simulink model "Adaptive_cruise_control_01"  (R2020a)
settings: Solver=VariableStepAuto  StartTime=0.0  StopTime=100  RelTol=1e-3
libraries: simulink x4, vrlib x2, mpcadaslib x1, robotmobilelib x1, autolibshared x1
settings Model: Creator=NIKHIL  LastModifiedBy=NIKHIL

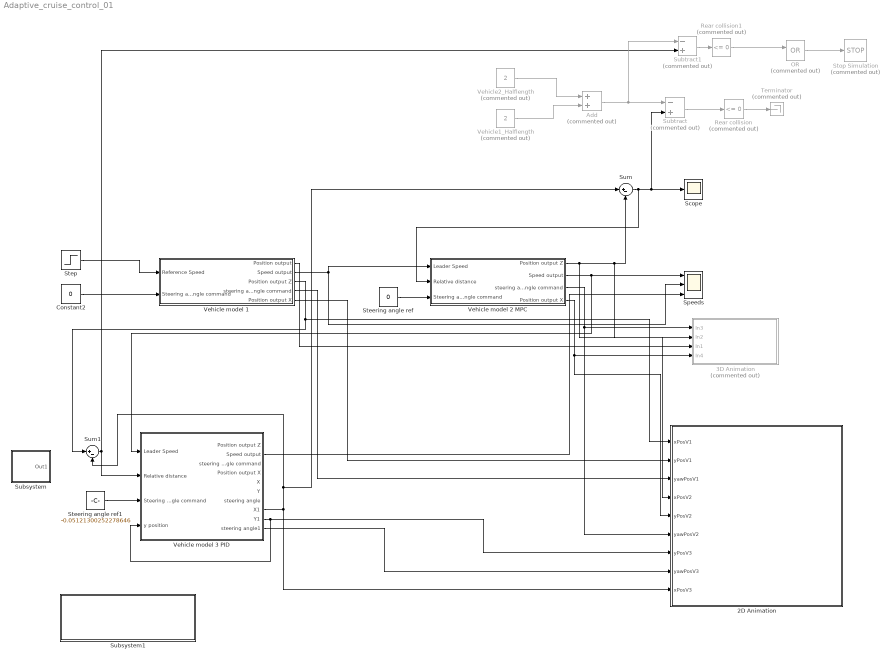
== system Adaptive_cruise_control_01 ==
  2D Animation : Subsystem  TreatAsAtomicUnit=on  SystemSampleTime=0.02
  3D Animation : Subsystem  Commented=on
  Add : Sum  Commented=on
  Constant2 : Constant  Value=0
  OR : Logic  Commented=on  Operator=OR  IconShape=distinctive  AllPortsSameDT=off  OutDataTypeStr=boolean
  Rear collision : simulink/Logic and Bit Operations/Compare To Constant  Commented=on  relop=<=  const=0  OutDataTypeStr=boolean
  Rear collision1 : simulink/Logic and Bit Operations/Compare To Constant  Commented=on  relop=<=  const=0  OutDataTypeStr=boolean
  Scope : Scope
  "Speeds " : Scope  NumInputPorts=3
  Steering angle ref : Constant  Value=0
  Steering angle ref1 : Constant  Value=-0.05121300252278646
  Step : Step  Time=10.5  Before=8  After=8  SampleTime=0
  Stop Simulation : Stop  Commented=on
  Subsystem : Subsystem
  Subsystem1 : Subsystem
  Subtract : Sum  Commented=on  Inputs=-+
  Subtract1 : Sum  Commented=on  Inputs=-+
  Sum : Sum  Inputs=|+-
  Sum1 : Sum  Inputs=|+-
  Terminator : Terminator  Commented=on
  Vehicle model 1 : Subsystem  mask{Pos=10, Speed=25}
      mask prompts: Pos "Initial position"; Speed "Initial speed"
      mask TypeOptions Pos: Initial position Z/Value
      mask TypeOptions Speed: Initial speed/Value
  Vehicle model 2 MPC : Subsystem  mask{Pos=50, Speed=25}
      mask prompts: Pos "Initial position"; Speed "Initial speed"
      mask TypeOptions Pos: Initial position Z/Value
      mask TypeOptions Speed: Initial speed/Value
  Vehicle model 3 PID : Subsystem  mask{Pos=0, Speed=45}
      mask prompts: Pos "Initial position"; Speed "Initial speed"
      mask TypeOptions Pos: Initial position Z/Value
      mask TypeOptions Speed: Initial speed/Value
  Vehicle1_Halflength : Constant  Commented=on  Value=2
  Vehicle2_Halflength : Constant  Commented=on  Value=2
  wires:
  Vehicle model 2 MPC/3(steering angle command) -> 2D Animation/6(yawPosV2), 3D Animation/1(In3)
  Sum1/1 -> Vehicle model 3 PID/2(Relative distance), Subtract1/2
  Subtract1/1 -> Rear collision1/1
  Vehicle model 3 PID/9(Y1) -> Vehicle model 3 PID/4(y position), 2D Animation/7(yPosV3)
  Subtract/1 -> Rear collision/1
  Vehicle model 3 PID/2(Speed output) -> "Speeds "/3
  Vehicle model 3 PID/8(X1) -> Sum/1, Sum1/2, 2D Animation/9(xPosV3)
  Vehicle model 3 PID/10(steering angle1) -> 2D Animation/8(yawPosV3)
  Sum/1 -> Vehicle model 2 MPC/2(Relative distance), Subtract/2, Scope/1
  Steering angle ref/1 -> Vehicle model 2 MPC/3(Steering angle command)
  Vehicle model 2 MPC/2(Speed output) -> Vehicle model 3 PID/1(Leader Speed), "Speeds "/1
  OR/1 -> Stop Simulation/1
  Vehicle model 2 MPC/1(Position output Z) -> 2D Animation/4(xPosV2), Sum/2, 3D Animation/2(In2)
  Add/1 -> Subtract1/1, Subtract/1
  Vehicle2_Halflength/1 -> Add/1
  Vehicle model 1/1(Position output) -> 3D Animation/3(In1)
  Vehicle1_Halflength/1 -> Add/2
  Vehicle model 1/2(Speed output) -> "Speeds "/2, Vehicle model 2 MPC/1(Leader Speed)
  Vehicle model 2 MPC/4(Position output X) -> 2D Animation/5(yPosV2), 3D Animation/4(In4)
  Constant2/1 -> Vehicle model 1/2(Steering angle command)
  Vehicle model 1/3(Position output Z) -> 2D Animation/1(xPosV1), Sum1/1
  Steering angle ref1/1 -> Vehicle model 3 PID/3(Steering angle command)
  Rear collision1/1 -> OR/1
  Rear collision/1 -> Terminator/1
  Vehicle model 1/5(Position output X) -> 2D Animation/2(yPosV1)
  Vehicle model 1/4(steering angle command) -> 2D Animation/3(yawPosV1)
  Step/1 -> Vehicle model 1/1(Reference Speed)

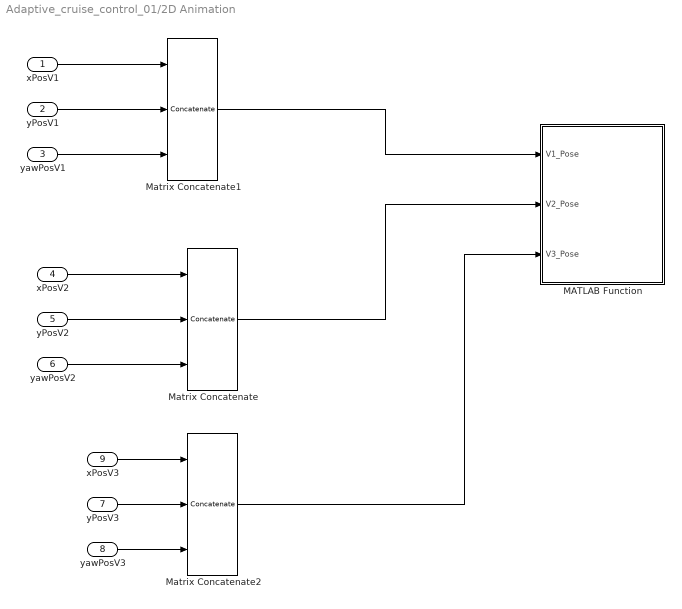
== system Adaptive_cruise_control_01/2D Animation ==
  xPosV1 : Inport
  yPosV1 : Inport  Port=2
  yawPosV1 : Inport  Port=3
  xPosV2 : Inport  Port=4
  yPosV2 : Inport  Port=5
  yawPosV2 : Inport  Port=6
  yPosV3 : Inport  Port=7
  yawPosV3 : Inport  Port=8
  xPosV3 : Inport  Port=9
  MATLAB Function : MATLAB Function  TreatAsAtomicUnit=on
      mask init:
      | close all;
      | figure('units','normalized','outerposition',[0 0 1 1]);
      | grid on
      | axis equal
      | hold on
  Matrix Concatenate : Concatenate  NumInputs=3  ConcatenateDimension=2
  Matrix Concatenate1 : Concatenate  NumInputs=3  ConcatenateDimension=2
  Matrix Concatenate2 : Concatenate  NumInputs=3  ConcatenateDimension=2
  wires:
  xPosV2/1 -> Matrix Concatenate/1
  yPosV2/1 -> Matrix Concatenate/2
  yawPosV2/1 -> Matrix Concatenate/3
  Matrix Concatenate/1 -> MATLAB Function/2(V2_Pose)
  xPosV1/1 -> Matrix Concatenate1/1
  yPosV1/1 -> Matrix Concatenate1/2
  yawPosV1/1 -> Matrix Concatenate1/3
  Matrix Concatenate1/1 -> MATLAB Function/1(V1_Pose)
  xPosV3/1 -> Matrix Concatenate2/1
  yPosV3/1 -> Matrix Concatenate2/2
  yawPosV3/1 -> Matrix Concatenate2/3
  Matrix Concatenate2/1 -> MATLAB Function/3(V3_Pose)

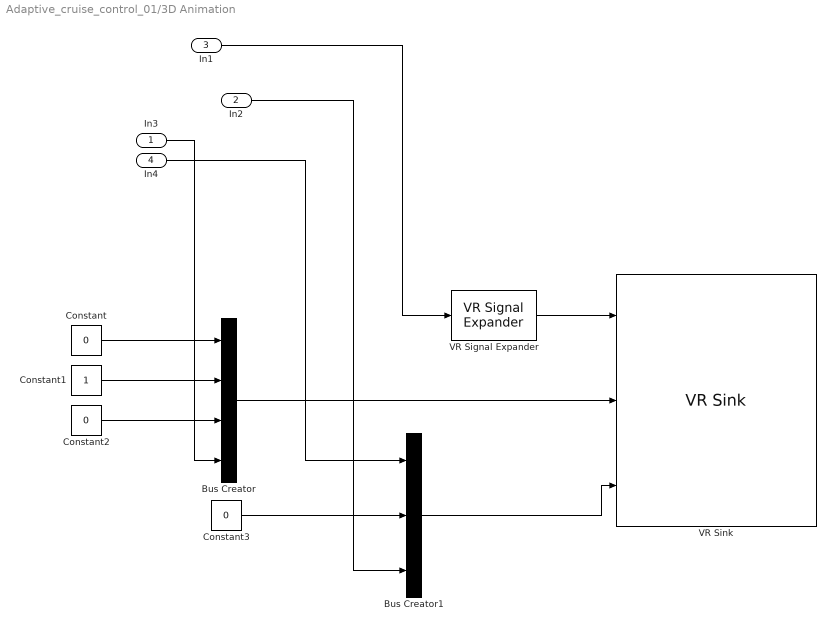
== system Adaptive_cruise_control_01/3D Animation ==
  In3 : Inport
  In2 : Inport  Port=2
  In1 : Inport  Port=3
  In4 : Inport  Port=4
  Bus Creator : BusCreator  Inputs=4
  Bus Creator1 : BusCreator  Inputs=3
  Constant : Constant  Value=0
  Constant1 : Constant
  Constant2 : Constant  Value=0
  Constant3 : Constant  Value=0
  VR Signal Expander : vrlib/VR Signal Expander  outwidth=3  outidx=[3]
  VR Sink : vrlib/VR Sink  InstantiateOnLoad=on  SampleTime=0.02  ViewEnable=on  RemoteChange=off  RemoteView=off  FieldsWritten=Car_Red.translation.3.1.1.double#Car_Blue.rotation.4.1.1.double#Car_Blue.translation.3.1.1.double  WorldFileName=PlatoonWorld.WRL  AutoView=off  VideoDimensions=[]  AllowVariableSize=off
  wires:
  In2/1 -> Bus Creator1/3
  Constant2/1 -> Bus Creator/3
  VR Signal Expander/1 -> VR Sink/1
  Bus Creator/1 -> VR Sink/2
  Constant1/1 -> Bus Creator/2
  Constant/1 -> Bus Creator/1
  Bus Creator1/1 -> VR Sink/3
  In4/1 -> Bus Creator1/1
  Constant3/1 -> Bus Creator1/2
  In1/1 -> VR Signal Expander/1
  In3/1 -> Bus Creator/4

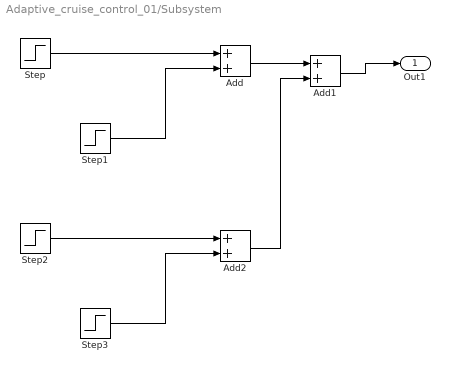
== system Adaptive_cruise_control_01/Subsystem ==
  Add : Sum
  Add1 : Sum
  Add2 : Sum
  Step : Step  Time=0  After=0.2  SampleTime=0
  Step1 : Step  After=-0.2  SampleTime=0
  Step2 : Step  Time=5  After=-0.12  SampleTime=0
  Step3 : Step  Time=6  After=0.12  SampleTime=0
  Out1 : Outport
  wires:
  Add/1 -> Add1/1
  Step/1 -> Add/1
  Step1/1 -> Add/2
  Step3/1 -> Add2/2
  Step2/1 -> Add2/1
  Add2/1 -> Add1/2
  Add1/1 -> Out1/1

== system Adaptive_cruise_control_01/Subsystem1 ==
  Dashboard Scope : DashboardScope
  Gauge : CircularGaugeBlock
  Knob : KnobBlock  ScaleMin=-0.2  ScaleMax=0.2

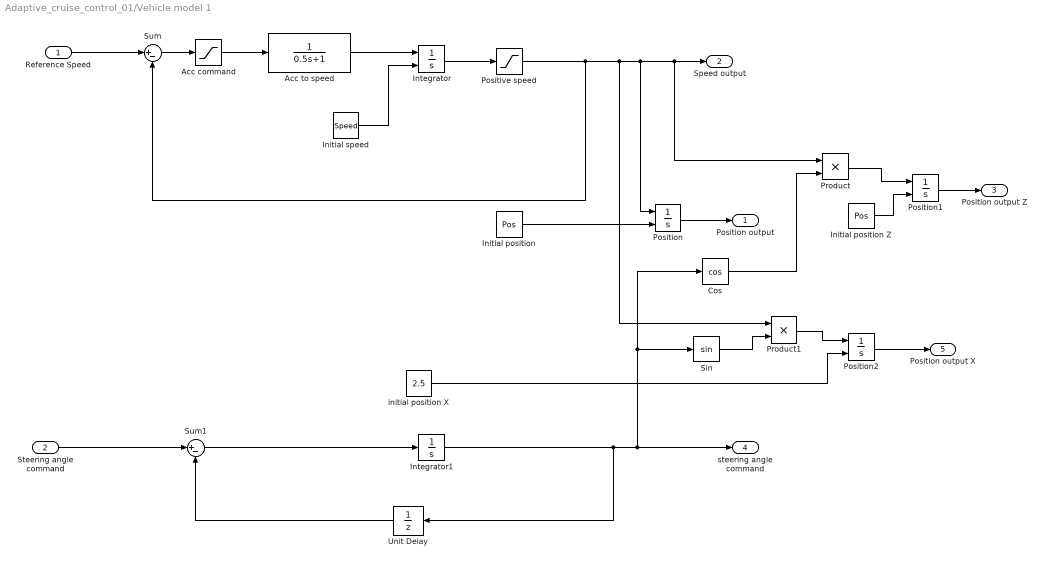
== system Adaptive_cruise_control_01/Vehicle model 1 ==
  Reference Speed : Inport
  Steering angle command : Inport  Port=2
  Acc command : Saturate  UpperLimit=2  LowerLimit=-3
  Acc to speed : TransferFcn  Denominator=[0.5 1]
  Cos : Trigonometry  Operator=cos
  Initial position : Constant  Value=Pos
  Initial position Z : Constant  Value=Pos
  Initial speed : Constant  Value=Speed
  Integrator : Integrator  InitialConditionSource=external
  Integrator1 : Integrator
  Position : Integrator  InitialConditionSource=external
  Position1 : Integrator  InitialConditionSource=external
  Position2 : Integrator  InitialConditionSource=external
  Positive speed : Saturate  UpperLimit=inf
  Product : Product
  Product1 : Product
  Sin : Trigonometry
  Sum : Sum  Inputs=|+-
  Sum1 : Sum  Inputs=|+-
  Unit Delay : UnitDelay  SampleTime=-1  HasFrameUpgradeWarning=on
  initial position X : Constant  Value=2.5
  Position output : Outport
  Speed output : Outport  Port=2
  Position output Z : Outport  Port=3
  steering angle command : Outport  Port=4
  Position output X : Outport  Port=5
  wires:
  Initial speed/1 -> Integrator/2
  Initial position/1 -> Position/2
  Sum/1 -> Acc command/1
  Integrator/1 -> Positive speed/1
  Acc to speed/1 -> Integrator/1
  Acc command/1 -> Acc to speed/1
  Position/1 -> Position output/1
  Reference Speed/1 -> Sum/1
  Cos/1 -> Product/2
  Initial position Z/1 -> Position1/2
  Product/1 -> Position1/1
  Position1/1 -> Position output Z/1
  Unit Delay/1 -> Sum1/2
  Position2/1 -> Position output X/1
  initial position X/1 -> Position2/2
  Sin/1 -> Product1/2
  Product1/1 -> Position2/1
  Integrator1/1 -> steering angle command/1, Sin/1, Cos/1, Unit Delay/1
  Steering angle command/1 -> Sum1/1
  Positive speed/1 -> Product1/1, Product/1, Speed output/1, Position/1, Sum/2
  Sum1/1 -> Integrator1/1

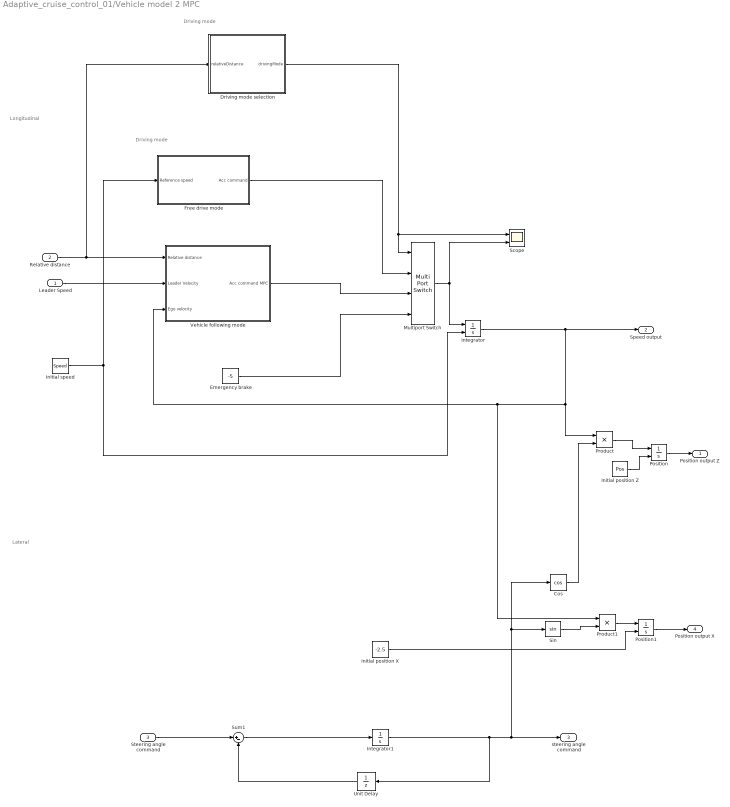
== system Adaptive_cruise_control_01/Vehicle model 2 MPC ==
  note: Driving mode
  note: Driving mode
  note: Lateral
  note: Longitudinal
  Leader Speed : Inport
  Relative distance : Inport  Port=2
  Steering angle command : Inport  Port=3
  Cos : Trigonometry  Operator=cos
  Driving mode selection : Stateflow chart  TreatAsAtomicUnit=on
  Emergency brake : Constant  Value=-5
  Free drive mode : Subsystem
  Initial position Z : Constant  Value=Pos
  Initial speed : Constant  Value=Speed
  Integrator : Integrator  InitialConditionSource=external  LimitOutput=on  LowerSaturationLimit=0
  Integrator1 : Integrator
  Multiport Switch : MultiPortSwitch
  Position : Integrator  InitialConditionSource=external
  Position1 : Integrator  InitialConditionSource=external
  Product : Product
  Product1 : Product
  Scope : Scope  NumInputPorts=2
  Sin : Trigonometry
  Sum1 : Sum  Inputs=|+-
  Unit Delay : UnitDelay  SampleTime=-1  HasFrameUpgradeWarning=on
  Vehicle following mode : Subsystem
  initial position X : Constant  Value=-2.5
  Position output Z : Outport
  Speed output : Outport  Port=2
  steering angle command : Outport  Port=3
  Position output X : Outport  Port=4
  wires:
  Position/1 -> Position output Z/1
  Initial position Z/1 -> Position/2
  Initial speed/1 -> Free drive mode/1(Reference speed), Integrator/2
  Integrator/1 -> Product/1, Vehicle following mode/3(Ego velocity), Product1/1, Speed output/1
  Steering angle command/1 -> Sum1/1
  Sum1/1 -> Integrator1/1
  Integrator1/1 -> Sin/1, Cos/1, steering angle command/1, Unit Delay/1
  Unit Delay/1 -> Sum1/2
  Cos/1 -> Product/2
  Product/1 -> Position/1
  initial position X/1 -> Position1/2
  Sin/1 -> Product1/2
  Product1/1 -> Position1/1
  Position1/1 -> Position output X/1
  Leader Speed/1 -> Vehicle following mode/2(Leader Velocity)
  Free drive mode/1(Acc command) -> Multiport Switch/2
  Multiport Switch/1 -> Scope/2, Integrator/1
  Driving mode selection/1(drivingMode) -> Multiport Switch/1, Scope/1
  Emergency brake/1 -> Multiport Switch/4
  Vehicle following mode/1(Acc command MPC) -> Multiport Switch/3
  Relative distance/1 -> Driving mode selection/1(relativeDistance), Vehicle following mode/1(Relative distance)

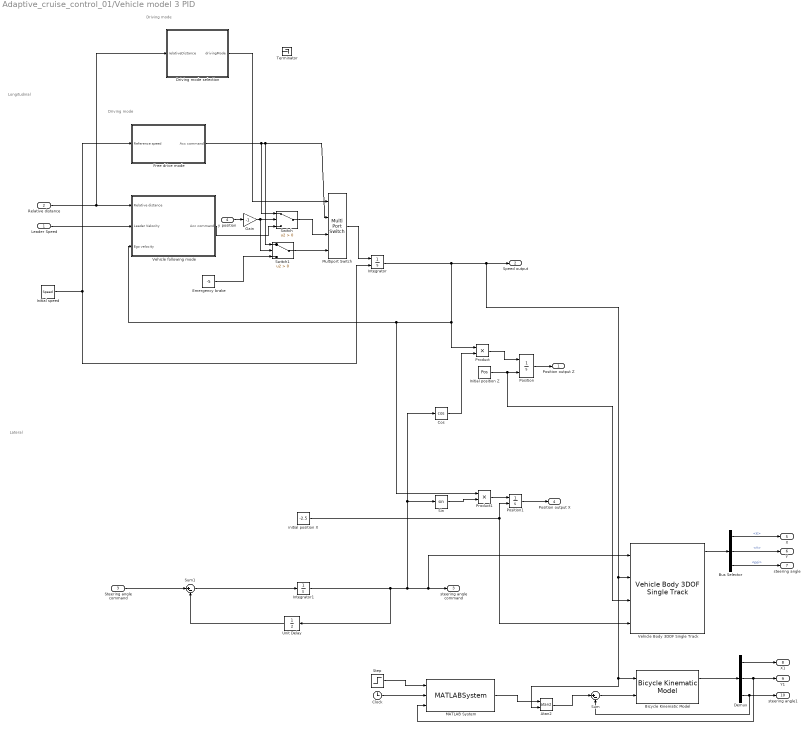
== system Adaptive_cruise_control_01/Vehicle model 3 PID ==
  note: Longitudinal
  note: Lateral
  note: Driving mode
  note: Driving mode
  Leader Speed : Inport
  Relative distance : Inport  Port=2
  Steering angle command : Inport  Port=3
  y position : Inport  Port=4
  Atan2 : Trigonometry  Operator=atan2
  Bicycle Kinematic Model : robotmobilelib/Bicycle Kinematic Model  VehicleInputs=Vehicle Speed & Steering Angle  WheelBase=3  VehicleSpeedRange=[0 12]  MaxSteeringAngle=pi/4  InitialState=[0; -2.5; 0]  SimulateUsing=Interpreted execution
      settings: SourceProductBaseCode=RO
  Bus Selector : BusSelector  OutputSignals=InertFrm.Cg.Disp.X,InertFrm.Cg.Disp.Y,InertFrm.Cg.Ang.psi
  Clock : Clock
  Cos : Trigonometry  Operator=cos
  Demux : Demux  Outputs=3
  Driving mode selection : Stateflow chart  TreatAsAtomicUnit=on
  Emergency brake : Constant  Value=-5
  Free drive mode : Subsystem
  Gain : Gain  Gain=-1
  Initial position Z : Constant  Value=Pos
  Initial speed : Constant  Value=Speed
  Integrator : Integrator  InitialConditionSource=external  LimitOutput=on  UpperSaturationLimit=12  LowerSaturationLimit=0
  Integrator1 : Integrator
  MATLAB System : MATLABSystem  System=LaneChanger  SimulateUsing=Interpreted execution
      mask Type: LaneChanger
      mask Display:
      | disp('LaneChanger');
      | port_label('input',1,'flag');
      | port_label('input',2,'clock');
      | port_label('input',3,'y');
      | port_label('output',1,'latSpeed');
  Multiport Switch : MultiPortSwitch
  Position : Integrator  InitialConditionSource=external
  Position1 : Integrator  InitialConditionSource=external
  Product : Product
  Product1 : Product
  Sin : Trigonometry
  Step : Step  Time=3  SampleTime=0
  Sum : Sum  Inputs=|+-
  Sum1 : Sum  Inputs=|+-
  Switch : Switch  Criteria=u2 > Threshold
  Switch1 : Switch  Criteria=u2 > Threshold
  Terminator : Terminator
  Unit Delay : UnitDelay  SampleTime=-1  HasFrameUpgradeWarning=on
  Vehicle Body 3DOF Single Track : autolibshared/Vehicle Body 3DOF Single Track  trackMode=Single (bicycle)  inputMode=External longitudinal velocity  frontSteerMode=on  rearSteerMode=off  windMode=off  muMode=off  extFMode=off  extMMode=off  extXo=on  extpsio=off  extxdoto=off  extro=off  extYo=on  extTamb=off  extydoto=off  aMode=2  NF=2  NR=2  m=2000  a=1.4  b=1.6  h=0.35  X_o=0  xdot_o=0  CalphaMode=off  sigmaMode=on  d=0  w=[1.4,1.4]  Cy_f=12e3  Cy_r=11e3  sigma_f=.1  sigma_r=.1  alpha_f_brk=[-.1 .1]  Cy_f_data=[-9e3 9e3]  alpha_r_brk=[-.1 .1]  Cy_r_data=[-9e3 9e3]  Y_o=0  ydot_o=0  Izz=4000  psi_o=0  r_o=0  Af=2  Cd=.3  Cl=.1  Cpm=.1  beta_w=[0:0.01:0.3]  Cs=[0:0.03:0.9]  Cym=[0:0.01:0.3]  Pabs=101325  Tair=273  g=9.81  mu=1  xdot_tol=.01  Fznom=5000  Fxtire_sat=7e4  Fytire_sat=7e4  longOff=0  latOff=0  vertOff=0  wrapAng=off
      settings: SourceProductBaseCode=PW,MT,VE,VP
  Vehicle following mode : Subsystem
  initial position X : Constant  Value=-2.5
  Position output Z : Outport
  Speed output : Outport  Port=2
  steering angle command : Outport  Port=3
  Position output X : Outport  Port=4
  X : Outport  Port=5
  Y : Outport  Port=6
  steering angle : Outport  Port=7
  X1 : Outport  Port=8
  Y1 : Outport  Port=9
  steering angle1 : Outport  Port=10
  wires:
  Multiport Switch/1 -> Integrator/1
  Leader Speed/1 -> Vehicle following mode/2(Leader Velocity)
  Position1/1 -> Position output X/1
  Product1/1 -> Position1/1
  Sin/1 -> Product1/2
  initial position X/1 -> Vehicle Body 3DOF Single Track/4, Position1/2
  Product/1 -> Position/1
  Cos/1 -> Product/2
  Unit Delay/1 -> Sum1/2
  Integrator1/1 -> Unit Delay/1, Vehicle Body 3DOF Single Track/1, steering angle command/1, Cos/1, Sin/1
  Sum1/1 -> Integrator1/1
  Steering angle command/1 -> Sum1/1
  Initial speed/1 -> Integrator/2, Free drive mode/1(Reference speed)
  Initial position Z/1 -> Vehicle Body 3DOF Single Track/3, Position/2
  Position/1 -> Position output Z/1
  Integrator/1 -> Atan2/2, Bicycle Kinematic Model/1, Vehicle Body 3DOF Single Track/2, Speed output/1, Product1/1, Vehicle following mode/3(Ego velocity), Product/1
  Vehicle Body 3DOF Single Track/1 -> Bus Selector/1
  Bus Selector/2 -> Y/1  "<Y>"
  Bus Selector/3 -> steering angle/1  "<psi>"
  Bus Selector/1 -> X/1  "<X>"
  Bicycle Kinematic Model/1 -> Demux/1
  Demux/2 -> MATLAB System/3, Y1/1
  Demux/1 -> X1/1
  Demux/3 -> Sum/2, steering angle1/1
  Step/1 -> MATLAB System/1
  Clock/1 -> MATLAB System/2
  MATLAB System/1 -> Atan2/1
  Atan2/1 -> Sum/1
  Sum/1 -> Bicycle Kinematic Model/2
  Driving mode selection/1(drivingMode) -> Multiport Switch/1
  y position/1 -> Gain/1
  Switch/1 -> Multiport Switch/3
  Switch1/1 -> Multiport Switch/4
  Free drive mode/1(Acc command) -> Switch/1, Multiport Switch/2, Switch1/1
  Relative distance/1 -> Driving mode selection/1(relativeDistance), Vehicle following mode/1(Relative distance)
  Gain/1 -> Switch1/2, Switch/2
  Vehicle following mode/1(Acc command) -> Switch/3
  Emergency brake/1 -> Switch1/3

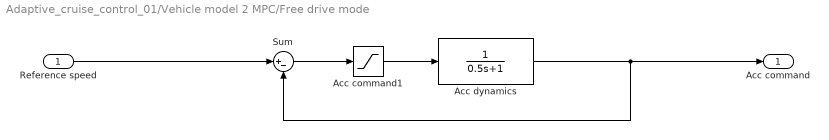
== system Adaptive_cruise_control_01/Vehicle model 2 MPC/Free drive mode ==
  Reference speed : Inport
  Acc command1 : Saturate  UpperLimit=2  LowerLimit=-3
  Acc dynamics : TransferFcn  Denominator=[0.5 1]
  Sum : Sum  Inputs=|+-
  Acc command : Outport
  wires:
  Sum/1 -> Acc command1/1
  Reference speed/1 -> Sum/1
  Acc dynamics/1 -> Sum/2, Acc command/1
  Acc command1/1 -> Acc dynamics/1

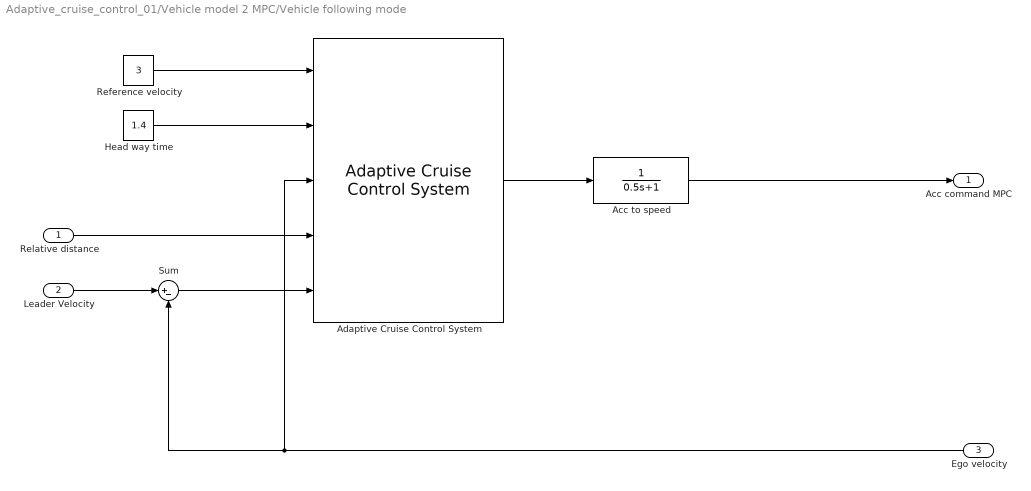
== system Adaptive_cruise_control_01/Vehicle model 2 MPC/Vehicle following mode ==
  Relative distance : Inport
  Leader Velocity : Inport  Port=2
  Ego velocity : Inport  Port=3
  Acc to speed : TransferFcn  Denominator=[0.5 1]
  Adaptive Cruise Control System : mpcadaslib/Adaptive Cruise Control System  EgoModel=tf(1,[0.5,1,0])  InitialEgoVelocity=30  DefaultSpacing=10  MaxVelocity=50  MinAcceleration=-3  amin_ext=off  MaxAcceleration=2  amax_ext=off  Ts=0.5  PredictionHorizon=200  ControllerBehavior=0.590  suboptimal=off  maxiter=10  datatypeopt=double  optmode=off  trackmode=off
  Head way time : Constant  Value=1.4
  Reference velocity : Constant  Value=3
  Sum : Sum  Inputs=|+-
  Acc command MPC : Outport
  wires:
  Acc to speed/1 -> Acc command MPC/1
  Relative distance/1 -> Adaptive Cruise Control System/4
  Ego velocity/1 -> Adaptive Cruise Control System/3, Sum/2
  Adaptive Cruise Control System/1 -> Acc to speed/1
  Leader Velocity/1 -> Sum/1
  Sum/1 -> Adaptive Cruise Control System/5
  Reference velocity/1 -> Adaptive Cruise Control System/1
  Head way time/1 -> Adaptive Cruise Control System/2

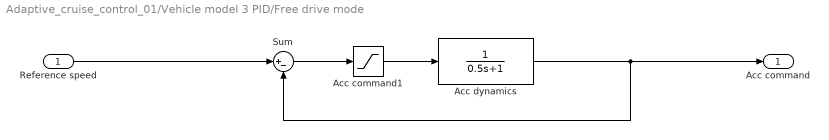
== system Adaptive_cruise_control_01/Vehicle model 3 PID/Free drive mode ==
  Reference speed : Inport
  Acc command1 : Saturate  UpperLimit=2  LowerLimit=-3
  Acc dynamics : TransferFcn  Denominator=[0.5 1]
  Sum : Sum  Inputs=|+-
  Acc command : Outport
  wires:
  Acc command1/1 -> Acc dynamics/1
  Acc dynamics/1 -> Acc command/1, Sum/2
  Reference speed/1 -> Sum/1
  Sum/1 -> Acc command1/1

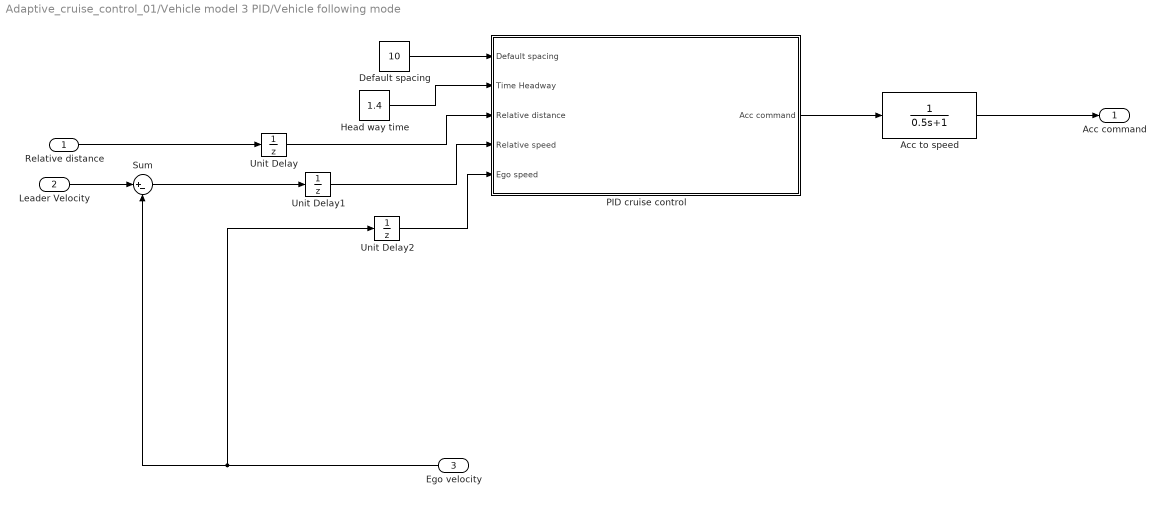
== system Adaptive_cruise_control_01/Vehicle model 3 PID/Vehicle following mode ==
  Relative distance : Inport
  Leader Velocity : Inport  Port=2
  Ego velocity : Inport  Port=3
  Acc to speed : TransferFcn  Denominator=[0.5 1]
  Default spacing : Constant  Value=10
  Head way time : Constant  Value=1.4
  PID cruise control : Subsystem
  Sum : Sum  Inputs=|+-
  Unit Delay : UnitDelay  SampleTime=-1  HasFrameUpgradeWarning=on
  Unit Delay1 : UnitDelay  SampleTime=-1  HasFrameUpgradeWarning=on
  Unit Delay2 : UnitDelay  SampleTime=-1  HasFrameUpgradeWarning=on
  Acc command : Outport
  wires:
  Sum/1 -> Unit Delay1/1
  Leader Velocity/1 -> Sum/1
  PID cruise control/1(Acc command) -> Acc to speed/1
  Ego velocity/1 -> Unit Delay2/1, Sum/2
  Relative distance/1 -> Unit Delay/1
  Acc to speed/1 -> Acc command/1
  Default spacing/1 -> PID cruise control/1(Default spacing)
  Unit Delay/1 -> PID cruise control/3(Relative distance)
  Unit Delay1/1 -> PID cruise control/4(Relative speed)
  Head way time/1 -> PID cruise control/2(Time Headway)
  Unit Delay2/1 -> PID cruise control/5(Ego speed)

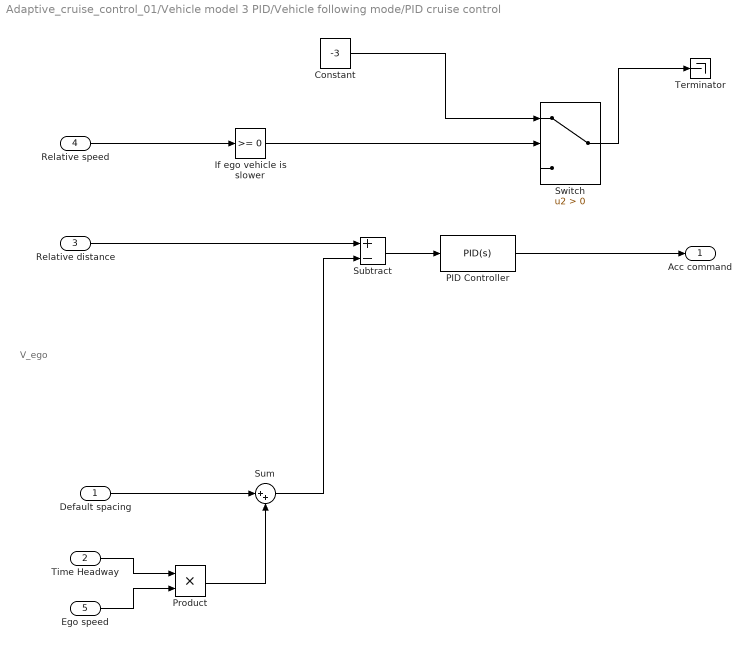
== system Adaptive_cruise_control_01/Vehicle model 3 PID/Vehicle following mode/PID cruise control ==
  note: V_ego
  Default spacing : Inport
  Time Headway : Inport  Port=2
  Relative distance : Inport  Port=3
  Relative speed : Inport  Port=4
  Ego speed : Inport  Port=5
  Constant : Constant  Value=-3
  If ego vehicle is slower : simulink/Logic and Bit Operations/Compare To Constant  relop=>=  const=0  OutDataTypeStr=boolean
  PID Controller : simulink/Continuous/PID Controller  Controller=PID  Form=Parallel  TimeDomain=Continuous-time  UseExternalTs=off  SampleTime=-1  IntegratorMethod=Forward Euler  FilterMethod=Forward Euler  ControllerParametersSource=internal  P=2  I=0.04  D=1.2  UseFilter=on  N=240  TunerSelectOption=Transfer Function Based (PID Tuner App)  InitialConditionSource=internal  InitialConditionForIntegrator=0  InitialConditionForFilter=0  DifferentiatorICPrevScaledInput=0  ExternalReset=none  TrackingMode=off  Kt=1  LimitOutput=on  UpperSaturationLimit=2  LowerSaturationLimit=-3  LinearizeAsGain=on  AntiWindupMode=clamping  Kb=1  POutMin=[]  POutMax=[]  IOutMin=[]  IOutMax=[]  DOutMin=[]  DOutMax=[]  NOutMin=[]  NOutMax=[]  SumOutMin=[]  SumOutMax=[]  SaturationOutMin=[]  SaturationOutMax=[]  PParamMin=[]  PParamMax=[]  IParamMin=[]  IParamMax=[]  DParamMin=[]  DParamMax=[]  NParamMin=[]  NParamMax=[]  KbParamMin=[]  KbParamMax=[]  KtParamMin=[]  KtParamMax=[]  KbOutMin=[]  KbOutMax=[]  KtOutMin=[]  KtOutMax=[]  IntegratorOutMin=[]  IntegratorOutMax=[]  FilterOutMin=[]  FilterOutMax=[]  SumI1OutMin=[]  SumI1OutMax=[]  SumI2OutMin=[]  SumI2OutMax=[]  SumI3OutMin=[]  SumI3OutMax=[]  SumI4OutMin=[]  SumI4OutMax=[]  SumDOutMin=[]  SumDOutMax=[]  DifferentiatorOutMin=[]  DifferentiatorOutMax=[]  FilterDiffOutCoefMin=[]  FilterDiffOutCoefMax=[]  ReciprocalOutMin=[]  ReciprocalOutMax=[]  SumDenOutMin=[]  SumDenOutMax=[]  SumNumOutMin=[]  SumNumOutMax=[]  DivideOutMin=[]  DivideOutMax=[]  UdiffTsProdOutMin=[]  UdiffTsProdOutMax=[]  NTsProdOutMin=[]  NTsProdOutMax=[]  UintegralTsProdOutMin=[]  UintegralTsProdOutMax=[]  UngainTsProdOutMin=[]  UngainTsProdOutMax=[]  IntegratorContinuousStateAttributes=''  IntegratorStateMustResolveToSignalObject=off  IntegratorRTWStateStorageClass=Auto  FilterContinuousStateAttributes=''  FilterStateMustResolveToSignalObject=off  FilterRTWStateStorageClass=Auto  ParallelPVariant=InternalParameters  IdealPVariant=Disabled  IVariant=InternalParameters  DVariant=InternalParameters  IntegratorVariant=Continuous  SatVariant=Enabled  AWVariant=ContClampingParallel  PCopyVariant=Disabled  TRVariant=Disabled  FdbkBlocksVariant=Forward  IdealPFdbkVariant=Disabled  SatFdbkVariant=Disabled  DerivativeFilterVariant=ContFilter  NVariant=InternalParameters  NCopyVariant=Disabled  FilterICVariant=InternalICsFilter  IntegratorICVariant=InternalICs  ExternalResetVariant=Disabled  TRSumVariant=Passthrough  SumFdbkVariant=Disabled  SumVariant=Sum_PID  TsampFilterVariant=InternalTs  TsampNgainVariant=Passthrough  TsampIntegralVariant=Passthrough
  Product : Product
  Subtract : Sum  Inputs=+-
  Sum : Sum  Inputs=|++
  Switch : Switch  Criteria=u2 > Threshold
  Terminator : Terminator
  Acc command : Outport
  wires:
  Time Headway/1 -> Product/1
  Ego speed/1 -> Product/2
  Default spacing/1 -> Sum/1
  Product/1 -> Sum/2
  Relative distance/1 -> Subtract/1
  Sum/1 -> Subtract/2
  Relative speed/1 -> If ego vehicle is slower/1
  If ego vehicle is slower/1 -> Switch/2
  Subtract/1 -> PID Controller/1
  Constant/1 -> Switch/1
  PID Controller/1 -> Acc command/1
  Switch/1 -> Terminator/1

== stateflow chart Adaptive_cruise_control_01/Vehicle model 3 PID/Driving mode selection ==
  state VehicleFollowing
    entry:
    drivingMode = 2;
  state FreeDrive
    entry:
    drivingMode = 1;
  state EmergencyBrake
    entry:
    drivingMode = 3;
  (default) -> FreeDrive
  VehicleFollowing -> FreeDrive [order 1] : [relativeDistance >50]
  FreeDrive -> VehicleFollowing [order 1] : [relativeDistance <=40]
  FreeDrive -> EmergencyBrake [order 2] : [relativeDistance <=10]
  EmergencyBrake -> VehicleFollowing : [relativeDistance >15]
  VehicleFollowing -> EmergencyBrake [order 2] : [relativeDistance <=10]
  data: relativeDistance input; drivingMode output

== matlab function Adaptive_cruise_control_01/2D Animation/MATLAB Function ==
  data: V1_Pose input; V2_Pose input; V3_Pose input
function plotVehicle(V1_Pose, V2_Pose, V3_Pose)
%% clear positon
cla;

 %% vehicle 1 pose
x1 = V1_Pose(1);
y1 = V1_Pose(2);
yaw1 = V1_Pose(3);

centerP=[x1;y1];

V1_HalfLength=2;
V1_HalfWidth=1;

% centering a rectangle
p1=[V1_HalfLength;V1_HalfWidth];
p2=[V1_HalfLength;-V1_HalfWidth];
p3=[-V1_HalfLength;-V1_HalfWidth];
p4=[-V1_HalfLength;V1_HalfWidth];

% rotating matrix
Rmatrix=[cos(yaw1) -sin(yaw1); sin(yaw1) cos(yaw1)];


% rotated point
p1r= centerP+Rmatrix*p1;
p2r= centerP+Rmatrix*p2;
p3r= centerP+Rmatrix*p3;
p4r= centerP+Rmatrix*p4;

%CONNECTING POINTS

Hitbox_V1=[p1r p2r p3r p4r p1r];

cornerV1_x=transpose(Hitbox_V1(1,:));
cornerV1_y=transpose(Hitbox_V1(2,:));


%% vehicle 2 pose
x2 = V2_Pose(1);
y2 = V2_Pose(2);
yaw2 = V2_Pose(3);

centerP=[x2;y2];

V2_HalfLength=2;
V2_HalfWidth=1;

% centering a rectangle
p1=[V2_HalfLength;V2_HalfWidth];
p2=[V2_HalfLength;-V2_HalfWidth];
p3=[-V2_HalfLength;-V2_HalfWidth];
p4=[-V2_HalfLength;V2_HalfWidth];

% rotating matrix
Rmatrix=[cos(yaw2) -sin(yaw2); sin(yaw2) cos(yaw2)];

% rotated point
p1r= centerP+Rmatrix*p1;
p2r= centerP+Rmatrix*p2;
p3r= centerP+Rmatrix*p3;
p4r= centerP+Rmatrix*p4;

%CONNECTING POINTS

Hitbox_V2=[p1r p2r p3r p4r p1r];

cornerV2_x=transpose(Hitbox_V2(1,:));
cornerV2_y=transpose(Hitbox_V2(2,:));

 %% vehicle 3 pose
 
x3 = V3_Pose(1);
y3 = V3_Pose(2);
yaw3 = V3_Pose(3);

centerP=[x3;y3];

V3_HalfLength=2;
V3_HalfWidth=1;

% centering a rectangle
p1=[V3_HalfLength;V3_HalfWidth];
p2=[V3_HalfLength;-V3_HalfWidth];
p3=[-V3_HalfLength;-V3_HalfWidth];
p4=[-V3_HalfLength;V3_HalfWidth];

% rotating matrix
Rmatrix=[cos(yaw3) -sin(yaw3); sin(yaw3) cos(yaw3)];


% rotated point
p1r= centerP+Rmatrix*p1;
p2r= centerP+Rmatrix*p2;
p3r= centerP+Rmatrix*p3;
p4r= centerP+Rmatrix*p4;

%CONNECTING POINTS

Hitbox_V3=[p1r p2r p3r p4r p1r];

cornerV3_x=transpose(Hitbox_V3(1,:));
cornerV3_y=transpose(Hitbox_V3(2,:));

%% plot vehicle
plot(cornerV1_x,cornerV1_y,'g'); % vehicle rectangle
plot(x1,y1,'* '); % vehicle center

plot(cornerV2_x,cornerV2_y,'r'); % vehicle rectangle
plot(x2,y2,'o'); % vehicle center

plot(cornerV3_x,cornerV3_y,'b'); % vehicle rectangle
plot(x3,y3,'x'); % vehicle center

upperLine=plot([0 1000], [5,5], 'color', 'blue');
midLine=plot([0 1000], [0,0], '--', 'color', 'blue');
upperLine=plot([0 1000], [-5,-5], 'color', 'blue');


% Adjust axis
axis([x3-40 x3+40 y3-20 y3+20]);

== stateflow chart Adaptive_cruise_control_01/Vehicle model 2 MPC/Driving mode selection ==
  state VehicleFollowing
    entry:
    drivingMode = 2;
  state FreeDrive
    entry:
    drivingMode = 1;
  state EmergencyBrake
    entry:
    drivingMode = 3;
  (default) -> FreeDrive
  VehicleFollowing -> FreeDrive [order 1] : [relativeDistance >50]
  FreeDrive -> VehicleFollowing [order 1] : [relativeDistance <=40]
  FreeDrive -> EmergencyBrake [order 2] : [relativeDistance <=10]
  EmergencyBrake -> VehicleFollowing : [relativeDistance >15]
  VehicleFollowing -> EmergencyBrake [order 2] : [relativeDistance <=10]
  data: relativeDistance input; drivingMode output
